simulink model "I_Control_and_G_Control_and_B_Control"  (R2024b)
settings: Solver=VariableStepAuto  StartTime=0.0  StopTime=time  RelTol=1e-3
values from neighbouring files (symbols this model uses):
  B = (y1-y4)/2    (= 0.75)    [Data.m]
  Cd = 0.28    [Data.m]
  dd = 2    [Data.m]
  delay_Pulse_time = 1.5    [Data.m]
  dk = 2    [Data.m]
  Fi = Ti/r    (= 156.25)    [Data.m]
  Fz = la/(la+lb)*m*g/2    (= 2450)    [Data.m]
  id = 0.01    [Data.m]
  ik = 1    [Data.m]
  Iw = 0.5    [Data.m]
  Iz = 1600    [Data.m]
  JL = 0.08    [Data.m]
  Jm = 6.96e-6    (= 6.96e-06)    [Data.m]
  Kb = 0.0525    [Data.m]
  Kf = 1.4e-3    (= 0.0014)    [Data.m]
  Km = 0.053    [Data.m]
  L = 6.2e-4    (= 0.00062)    [Data.m]    (also in submit.m = (1-nameda1)*(1-0.015*u1*sqrt((cx^2)*(nameda1^2)+(cy^2)*((tan)
  la = x1    (= 1.25)    [Data.m]
  lb = x1    (= 1.25)    [Data.m]
  m = 1000    [Data.m]
  n = 1/200    (= 0.005)    [Data.m]
  pd = 100    [Data.m]
  pk = 300    [Data.m]
  r = 0.32    [Data.m]
  R = 2.07    [Data.m]
  x1_fc = 0.01    [Data.m]
  x1_jz = 0    [Data.m]
  x2_fc = 0.05    [Data.m]
  x2_jz = 0.01    [Data.m]
  x3_fc = 0.1    [Data.m]
  x3_jz = 0.05    [Data.m]
  x4_fc = 0.5    [Data.m]
  x4_jz = 0.08    [Data.m]
  Xicr = 0,Yicr=10    [Data.m]
undefined symbols (not defined in the file or in its folder): Yicr
libraries: slpidlib x8
settings Model: Creator=hzh  LastModifiedBy=hzh
settings DataIOCC: ReturnWorkspaceOutputsName=out2
settings RTWCC: GPUComputeCapability=3.5

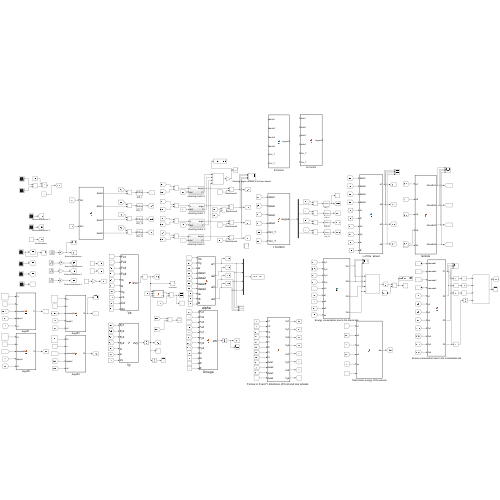
[thumbnail: Simulink's stored preview of the top-level diagram]
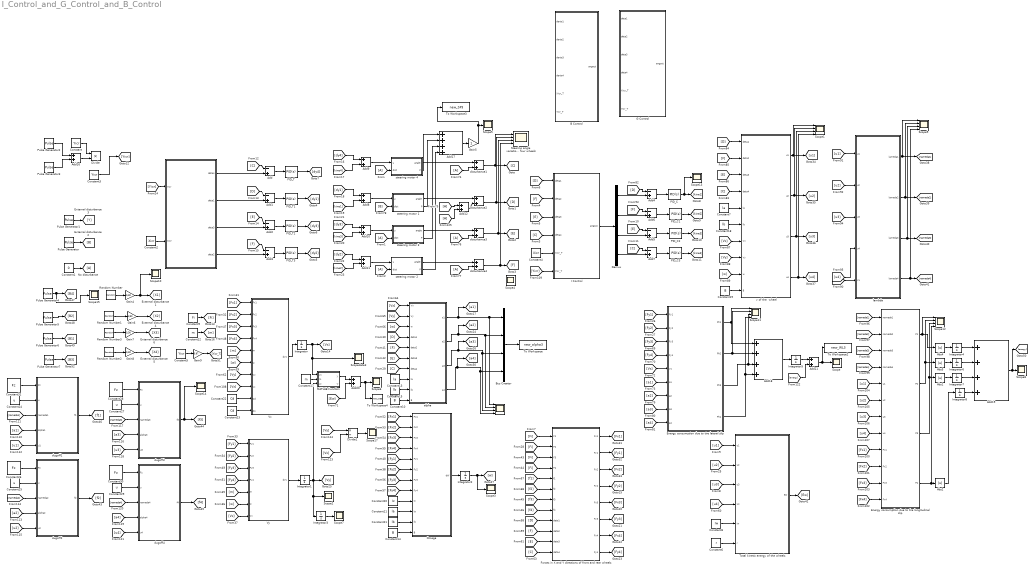
== system I_Control_and_G_Control_and_B_Control ==
  " " : MATLAB Function  TreatAsAtomicUnit=on
  "                    " : Scope  NumInputPorts=4
  Abs{1..2,4..5} (4 alike) : Abs  SaturateOnIntegerOverflow=off
  Add{,1..7} (8 alike) : Sum  Inputs=-+
  Add{8..12,16,20..21} (8 alike) : Sum
  Add17 : Sum  Inputs=++++
  Add18 : Sum  Inputs=++++
  Add19 : Sum  Inputs=++++
  B Control : MATLAB Function  TreatAsAtomicUnit=on
  Bus Creator : BusCreator  Inputs=4
  Constant : Constant  Value=Yicr
  Constant1 : Constant  Value=0
  Constant10 : Constant  Value=B
  Constant11 : Constant  Value=la
  Constant12 : Constant  Value=m
  Constant13 : Constant  Value=la
  Constant14 : Constant  Value=B
  Constant15 : Constant  Value=lb
  Constant17 : Constant  Value=m
  Constant18 : Constant  Value=lb
  Constant19 : Constant  Value=B
  Constant2 : Constant  Value=Xicr
  Constant20 : Constant  Value=Iz
  Constant21 : Constant  Value=lb
  Constant22 : Constant  Value=Cd
  Constant23 : Constant  Value=Cd
  Constant{24..25,27,29} (4 alike) : Constant  Value=u
  Constant{26,28,30..31} (4 alike) : Constant  Value=Fz
  Constant3 : Constant  Value=Yicr
  Constant4 : Constant  Value=Xicr
  Constant5 : Constant  Value=Yicr
  Constant6 : Constant  Value=r
  Constant7 : Constant  Value=la
  Constant8 : Constant  Value=Iw
  Constant9 : Constant  Value=Fi
  Demux : Demux
  Divide : Product  Inputs=**
  Divide1 : Product  Inputs=*/
  Energy consumption due to tire lateral slip : MATLAB Function  TreatAsAtomicUnit=on
  Energy consumption due to tire longitudinal slip : MATLAB Function  TreatAsAtomicUnit=on
  "Forces in X and Y directions of front and rear wheels  " : MATLAB Function  TreatAsAtomicUnit=on
  From{,1..2,74..77,125} (8 alike) : From
  G Control : MATLAB Function  TreatAsAtomicUnit=on
  Gain{4,6..8} (4 alike) : Gain  Gain=1/30
  Gain5 : Gain
  Gain9 : Gain  Gain=0.97
  I Control : MATLAB Function  TreatAsAtomicUnit=on
  Integrator : Integrator  InitialCondition=0.0001
  Integrator1 : Integrator
  Integrator2 : Integrator
  Integrator3 : Integrator
  Integrator{4..8} (5 alike) : Integrator  InitialCondition=0.01
  MATLAB Function : MATLAB Function  TreatAsAtomicUnit=on
  No disturbance : Goto
  Omega : MATLAB Function  TreatAsAtomicUnit=on
  PID_C{,1..3} (4 alike) : slpidlib/PID Controller  Controller=PID  Form=Parallel  TimeDomain=Continuous-time  UseExternalTs=off  SampleTime=-1  IntegratorMethod=Forward Euler  FilterMethod=Forward Euler  ControllerParametersSource=internal  P=pk  I=ik  UseKiTs=off  D=dk  UseExternalDerivativeSource=off  N=100  UseFilter=on  TunerSelectOption=Transfer Function Based (PID Tuner App)  InitialConditionSource=internal  InitialConditionForIntegrator=0  InitialConditionForFilter=0  DifferentiatorICPrevScaledInput=0  ExternalReset=none  TrackingMode=off  Kt=1  LimitOutput=off  SatLimitsSource=internal  UpperSaturationLimit=inf  LowerSaturationLimit=-inf  LinearizeAsGain=on  AntiWindupMode=none  Kb=1  LimitIntegrator=off  UpperIntegratorSaturationLimit=inf  LowerIntegratorSaturationLimit=-inf  POutMin=[]  POutMax=[]  IOutMin=[]  IOutMax=[]  DOutMin=[]  DOutMax=[]  NOutMin=[]  NOutMax=[]  SumOutMin=[]  SumOutMax=[]  SaturationOutMin=[]  SaturationOutMax=[]  PParamMin=[]  PParamMax=[]  IParamMin=[]  IParamMax=[]  DParamMin=[]  DParamMax=[]  NParamMin=[]  NParamMax=[]  KbParamMin=[]  KbParamMax=[]  KtParamMin=[]  KtParamMax=[]  KbOutMin=[]  KbOutMax=[]  KtOutMin=[]  KtOutMax=[]  IntegratorOutMin=[]  IntegratorOutMax=[]  FilterOutMin=[]  FilterOutMax=[]  SumI1OutMin=[]  SumI1OutMax=[]  SumI2OutMin=[]  SumI2OutMax=[]  SumI3OutMin=[]  SumI3OutMax=[]  SumI4OutMin=[]  SumI4OutMax=[]  SumDOutMin=[]  SumDOutMax=[]  DifferentiatorOutMin=[]  DifferentiatorOutMax=[]  FilterDiffOutCoefMin=[]  FilterDiffOutCoefMax=[]  ReciprocalOutMin=[]  ReciprocalOutMax=[]  SumDenOutMin=[]  SumDenOutMax=[]  SumNumOutMin=[]  SumNumOutMax=[]  DivideOutMin=[]  DivideOutMax=[]  UdiffTsProdOutMin=[]  UdiffTsProdOutMax=[]  NTsProdOutMin=[]  NTsProdOutMax=[]  UintegralTsProdOutMin=[]  UintegralTsProdOutMax=[]  UngainTsProdOutMin=[]  UngainTsProdOutMax=[]  ClampingZeroOutDataTypeStr=Inherit: Inherit via back propagation  ClampingZeroOutMin=[]  ClampingZeroOutMax=[]  FilterDenConstantOutDataTypeStr=Inherit: Inherit via back propagation  FilterDenConstantOutMin=[]  FilterDenConstantOutMax=[]  PCopyOutDataTypeStr=Inherit: Inherit via back propagation  PCopyOutMin=[]  PCopyOutMax=[]  NCopyOutDataTypeStr=Inherit: Inherit via back propagation  NCopyOutMin=[]  NCopyOutMax=[]  IntegratorContinuousStateAttributes=''  IntegratorStateMustResolveToSignalObject=off  IntegratorRTWStateStorageClass=Auto  FilterContinuousStateAttributes=''  FilterStateMustResolveToSignalObject=off  FilterRTWStateStorageClass=Auto  ParallelPVariant=InternalParameters  IdealPVariant=Disabled  IVariant=InternalParameters  DVariant=InternalParameters  IntegratorVariant=Continuous  SatVariant=Disabled  AWVariant=Passthrough  PCopyVariant=Disabled  TRVariant=Disabled  FdbkBlocksVariant=Forward  IdealPFdbkVariant=Disabled  SatFdbkVariant=Disabled  DerivativeFilterVariant=ContFilter  NVariant=InternalParameters  NCopyVariant=Disabled  FilterICVariant=InternalICsFilter  IntegratorICVariant=InternalICs  ExternalResetVariant=Disabled  TRSumVariant=Passthrough  SumFdbkVariant=Disabled  SumVariant=Sum_PID  TsampFilterVariant=InternalTs  TsampNgainVariant=Passthrough  TsampIntegralVariant=Disabled_SignalSpec  ExternalSaturationOutDataTypeStr=Inherit: Same as second input  DerivativeSourceVariant=ErrorSignal  PreIntVariant=InternalPreInt
  PID_T{,1..3} (4 alike) : slpidlib/PID Controller  Controller=PID  Form=Parallel  TimeDomain=Continuous-time  UseExternalTs=off  SampleTime=-1  IntegratorMethod=Forward Euler  FilterMethod=Forward Euler  ControllerParametersSource=internal  P=pd  I=id  UseKiTs=off  D=dd  UseExternalDerivativeSource=off  N=100  UseFilter=on  TunerSelectOption=Transfer Function Based (PID Tuner App)  InitialConditionSource=internal  InitialConditionForIntegrator=0  InitialConditionForFilter=0  DifferentiatorICPrevScaledInput=0  ExternalReset=none  TrackingMode=off  Kt=1  LimitOutput=off  SatLimitsSource=internal  UpperSaturationLimit=inf  LowerSaturationLimit=-inf  LinearizeAsGain=on  AntiWindupMode=none  Kb=1  LimitIntegrator=off  UpperIntegratorSaturationLimit=inf  LowerIntegratorSaturationLimit=-inf  POutMin=[]  POutMax=[]  IOutMin=[]  IOutMax=[]  DOutMin=[]  DOutMax=[]  NOutMin=[]  NOutMax=[]  SumOutMin=[]  SumOutMax=[]  SaturationOutMin=[]  SaturationOutMax=[]  PParamMin=[]  PParamMax=[]  IParamMin=[]  IParamMax=[]  DParamMin=[]  DParamMax=[]  NParamMin=[]  NParamMax=[]  KbParamMin=[]  KbParamMax=[]  KtParamMin=[]  KtParamMax=[]  KbOutMin=[]  KbOutMax=[]  KtOutMin=[]  KtOutMax=[]  IntegratorOutMin=[]  IntegratorOutMax=[]  FilterOutMin=[]  FilterOutMax=[]  SumI1OutMin=[]  SumI1OutMax=[]  SumI2OutMin=[]  SumI2OutMax=[]  SumI3OutMin=[]  SumI3OutMax=[]  SumI4OutMin=[]  SumI4OutMax=[]  SumDOutMin=[]  SumDOutMax=[]  DifferentiatorOutMin=[]  DifferentiatorOutMax=[]  FilterDiffOutCoefMin=[]  FilterDiffOutCoefMax=[]  ReciprocalOutMin=[]  ReciprocalOutMax=[]  SumDenOutMin=[]  SumDenOutMax=[]  SumNumOutMin=[]  SumNumOutMax=[]  DivideOutMin=[]  DivideOutMax=[]  UdiffTsProdOutMin=[]  UdiffTsProdOutMax=[]  NTsProdOutMin=[]  NTsProdOutMax=[]  UintegralTsProdOutMin=[]  UintegralTsProdOutMax=[]  UngainTsProdOutMin=[]  UngainTsProdOutMax=[]  ClampingZeroOutDataTypeStr=Inherit: Inherit via back propagation  ClampingZeroOutMin=[]  ClampingZeroOutMax=[]  FilterDenConstantOutDataTypeStr=Inherit: Inherit via back propagation  FilterDenConstantOutMin=[]  FilterDenConstantOutMax=[]  PCopyOutDataTypeStr=Inherit: Inherit via back propagation  PCopyOutMin=[]  PCopyOutMax=[]  NCopyOutDataTypeStr=Inherit: Inherit via back propagation  NCopyOutMin=[]  NCopyOutMax=[]  IntegratorContinuousStateAttributes=''  IntegratorStateMustResolveToSignalObject=off  IntegratorRTWStateStorageClass=Auto  FilterContinuousStateAttributes=''  FilterStateMustResolveToSignalObject=off  FilterRTWStateStorageClass=Auto  ParallelPVariant=InternalParameters  IdealPVariant=Disabled  IVariant=InternalParameters  DVariant=InternalParameters  IntegratorVariant=Continuous  SatVariant=Disabled  AWVariant=Passthrough  PCopyVariant=Disabled  TRVariant=Disabled  FdbkBlocksVariant=Forward  IdealPFdbkVariant=Disabled  SatFdbkVariant=Disabled  DerivativeFilterVariant=ContFilter  NVariant=InternalParameters  NCopyVariant=Disabled  FilterICVariant=InternalICsFilter  IntegratorICVariant=InternalICs  ExternalResetVariant=Disabled  TRSumVariant=Passthrough  SumFdbkVariant=Disabled  SumVariant=Sum_PID  TsampFilterVariant=InternalTs  TsampNgainVariant=Passthrough  TsampIntegralVariant=Disabled_SignalSpec  ExternalSaturationOutDataTypeStr=Inherit: Same as second input  DerivativeSourceVariant=ErrorSignal  PreIntVariant=InternalPreInt
  Pulse Generator : DiscretePulseGenerator  PulseType=Time based  Amplitude=(Pulse)  Period=100  PulseWidth=0.2  PhaseDelay=delay_Pulse_time
  Pulse Generator1 : DiscretePulseGenerator  PulseType=Time based  Amplitude=50  Period=100  PulseWidth=0.2  PhaseDelay=4
  Pulse Generator2 : DiscretePulseGenerator  PulseType=Time based  Period=5  PulseWidth=50
  Pulse Generator3 : DiscretePulseGenerator  PulseType=Time based  Amplitude=-1  Period=5  PulseWidth=50  PhaseDelay=2.5
  Pulse Generator4 : DiscretePulseGenerator  PulseType=Time based  Amplitude=0.16  Period=15  PulseWidth=15  PhaseDelay=12
  Pulse Generator5 : DiscretePulseGenerator  PulseType=Time based  Amplitude=0.1  Period=15  PulseWidth=5  PhaseDelay=8
  Pulse Generator6 : DiscretePulseGenerator  PulseType=Time based  Amplitude=0.05  Period=10  PulseWidth=5  PhaseDelay=4
  Pulse Generator7 : DiscretePulseGenerator  PulseType=Time based  Amplitude=0.2  Period=15  PulseWidth=4  PhaseDelay=1.5
  Random Number : RandomNumber  Mean=x1_jz  Variance=x1_fc  SampleTime=0.1
  Random Number1 : RandomNumber  Mean=x2_jz  Variance=x2_fc  SampleTime=0.1
  Random Number2 : RandomNumber  Mean=x4_jz  Variance=x4_fc  SampleTime=0.1
  Random Number3 : RandomNumber  Mean=x3_jz  Variance=x3_fc  SampleTime=0.1
  Scope{,2..3,5..8,10,13..15,17} (12 alike) : Scope
  Scope{1,9,11..12} (4 alike) : Scope  NumInputPorts=4
  Scope4 : Scope  NumInputPorts=2
  Scopedata3 : Scope
  Steering angle variation of the four wheels : Scope  NumInputPorts=4
  To Workspace : ToWorkspace  VariableName=new_alpha3  SampleTime=-1
  To Workspace2 : ToWorkspace  VariableName=new_WL3  SampleTime=-1
  To Workspace3 : ToWorkspace  VariableName=new_SP3  SampleTime=-1
  To Workspace4 : ToWorkspace  VariableName=new_KE3  SampleTime=-1
  Total kinetic energy of the wheels : MATLAB Function  TreatAsAtomicUnit=on
  Vx : MATLAB Function  TreatAsAtomicUnit=on
  Vy : MATLAB Function  TreatAsAtomicUnit=on
  alpha : MATLAB Function  TreatAsAtomicUnit=on
  disturbance{1..4} (4 alike) : Sum
  "dugoff1 " : MATLAB Function  TreatAsAtomicUnit=on
  dugoff2 : MATLAB Function  TreatAsAtomicUnit=on
  dugoff3 : MATLAB Function  TreatAsAtomicUnit=on
  dugoff4 : MATLAB Function  TreatAsAtomicUnit=on
  lambda : MATLAB Function  TreatAsAtomicUnit=on
  steering motor 1 : Subsystem
  steering motor 2 : Subsystem
  steering motor 3 : Subsystem
  steering motor 4 : Subsystem
  v of the  wheel : MATLAB Function  TreatAsAtomicUnit=on
  wires:
  Energy consumption due to tire longitudinal slip/2(P2) -> Abs5/1, Scope12/2
  " "/2(deta1) -> Add1/2
  [u3] -> Energy consumption due to tire longitudinal slip/7(u3)
  alpha/4(a4) -> [a4], "                    "/4, Bus Creator/4
  Integrator6/1 -> Add19/2
  " "/3(deta3) -> Add2/2
  [Fx4] -> Energy consumption due to tire longitudinal slip/12(Fx4)
  "Forces in X and Y directions of front and rear wheels  "/6(Fy3) -> [Fy3]
  Integrator8/1 -> Add19/4
  [Fx2] -> Energy consumption due to tire longitudinal slip/10(Fx2)
  Add6/1 -> PID_C1/1
  Abs4/1 -> Integrator4/1
  Demux/4 -> Add7/2
  Abs2/1 -> Integrator8/1
  Abs5/1 -> Integrator6/1
  [a4] -> Energy consumption due to tire lateral slip/9(a4)
  v of the  wheel/2(u2) -> Scope1/2, [u2]
  [Vx] -> alpha/1(Vx)
  [C] -> Add/1
  lambda/3(lameda3) -> [nameda3], Scope9/3
  [Fx3] -> Energy consumption due to tire longitudinal slip/11(Fx3)
  v of the  wheel/3(u3) -> Scope1/3, [u3]
  [Fi] -> "Forces in X and Y directions of front and rear wheels  "/1(F1)
  Energy consumption due to tire longitudinal slip/1(P1) -> Abs4/1, Scope12/1
  [a1] -> Energy consumption due to tire lateral slip/6(a1)
  Energy consumption due to tire longitudinal slip/3(P3) -> Abs1/1, Scope12/3
  From77/1 -> disturbance4/2
  Constant12/1 -> [m]
  Add18/1 -> Integrator5/1
  Add19/1 -> [energy], Scope8/1
  [u1] -> lambda/1(u1)
  Energy consumption due to tire lateral slip/4(Ph4) -> Add18/4, Scope11/4
  [u2] -> Energy consumption due to tire longitudinal slip/6(u2)
  [B] -> steering motor 1/2(dist)
  lambda/4(lameda4) -> Scope9/4, [nameda4]
  [nameda4] -> Energy consumption due to tire longitudinal slip/4(nameda4)
  [Vx] -> v of the  wheel/7(Vx)
  Energy consumption due to tire lateral slip/3(Ph3) -> Scope11/3, Add18/3
  lambda/2(lameda2) -> Scope9/2, [nameda2]
  [nameda2] -> Energy consumption due to tire longitudinal slip/2(nameda2)
  [w] -> Vx/6(w)
  Omega/1(dW) -> Integrator2/1
  Constant18/1 -> v of the  wheel/6(lb)
  Add11/1 -> steering motor 2/1(u)
  [a2] -> Energy consumption due to tire lateral slip/7(a2)
  [Fi] -> "Forces in X and Y directions of front and rear wheels  "/4(F4)
  steering motor 1/2(P) -> Add17/2
  [u4] -> lambda/4(u4)
  [F] -> v of the  wheel/2(deta2)
  Constant10/1 -> alpha/10(B)
  [kine4] -> Add9/2
  [u2] -> lambda/2(u2)
  Integrator7/1 -> Add19/3
  Integrator2/1 -> Scope3/1, [w]
  Constant7/1 -> v of the  wheel/5(la)
  [Yicr] -> " "/1(Yicr)
  [Vx] -> lambda/5(Vx)
  Energy consumption due to tire lateral slip/2(Ph2) -> Scope11/2, Add18/2
  [w] -> v of the  wheel/9(w)
  [D] -> v of the  wheel/1(deta1)
  [Vy] -> v of the  wheel/8(Vy)
  steering motor 4/2(P) -> Add17/1
  [a3] -> Energy consumption due to tire lateral slip/8(a3)
  PID_T3/1 -> [dy2]
  [Fy1] -> Energy consumption due to tire lateral slip/1(Fy1)
  [Fy3] -> Energy consumption due to tire lateral slip/3(Fy3)
  [Vx] -> Energy consumption due to tire lateral slip/5(Vx)
  [D] -> "Forces in X and Y directions of front and rear wheels  "/9(deta1)
  PID_C/1 -> Scope13/1, [kine1]
  Energy consumption due to tire lateral slip/1(Ph1) -> Scope11/1, Add18/1
  Integrator/1 -> [Vx], Scopedata3/1, MATLAB Function/1(vx)
  Constant2/1 -> " "/2(Xicr)
  [Fx1] -> Omega/1(Fx1)
  Add2/1 -> PID_T2/1
  "Forces in X and Y directions of front and rear wheels  "/3(Fx2) -> [Fx2]
  [f4] -> "Forces in X and Y directions of front and rear wheels  "/8(f4)
  Gain6/1 -> [X2]
  Constant13/1 -> alpha/8(la)
  [Fi] -> "Forces in X and Y directions of front and rear wheels  "/2(F2)
  Random Number3/1 -> Gain7/1
  Gain8/1 -> [X4]
  Gain7/1 -> [X3]
  [Fy2] -> Vy/2(Fy2)
  [u4] -> Energy consumption due to tire longitudinal slip/8(u4)
  Add17/1 -> Gain5/1
  [nameda3] -> Energy consumption due to tire longitudinal slip/3(nameda3)
  [Fy2] -> Omega/6(Fy2)
  [Fx2] -> Omega/2(Fx2)
  Random Number1/1 -> Gain6/1
  [E] -> v of the  wheel/3(deta3)
  Integrator3/1 -> Scope7/1
  Constant/1 -> Divide/1
  " "/1(deta4) -> Add/2
  PID_C2/1 -> [kine3]
  Add16/1 -> Divide/2
  From76/1 -> disturbance3/2
  [nameda1] -> Energy consumption due to tire longitudinal slip/1(nameda1)
  [D] -> Add4/1
  steering motor 2/1(angle) -> disturbance4/1
  v of the  wheel/1(u1) -> Scope1/1, [u1]
  PID_C1/1 -> [kine2]
  Gain5/1 -> To Workspace3/1, Scope5/1
  Constant20/1 -> Omega/9(Iz)
  [u3] -> lambda/3(u3)
  steering motor 2/2(P) -> Add17/4
  steering motor 3/2(P) -> Add17/3
  " "/4(deta2) -> Add3/2
  Demux/2 -> Add6/2
  Pulse Generator3/1 -> Add16/2
  [C] -> v of the  wheel/4(deta4)
  disturbance2/1 -> Steering angle variation of the four wheels/2, [D]
  disturbance3/1 -> Steering angle variation of the four wheels/3, [E]
  [Fx3] -> Vx/3(Fx3)
  [m] -> Vy/5(m)
  Integrator1/1 -> MATLAB Function/3(vy), Integrator3/1, Scope2/1, [Vy]
  Pulse Generator/1 -> [B]
  "Forces in X and Y directions of front and rear wheels  "/1(Fx1) -> [Fx1]
  Pulse Generator1/1 -> [Y]
  From74/1 -> disturbance1/2
  Constant11/1 -> Omega/10(la)
  [u1] -> Energy consumption due to tire longitudinal slip/5(u1)
  Random Number/1 -> Gain4/1
  [Fx4] -> Vx/4(Fx4)
  Vx/1(dVx) -> Integrator/1
  disturbance1/1 -> Steering angle variation of the four wheels/1, [C]
  "Forces in X and Y directions of front and rear wheels  "/5(Fx3) -> [Fx3]
  Vy/1(dVy) -> Integrator1/1
  Constant17/1 -> MATLAB Function/2(m)
  Gain4/1 -> Scope10/1, [X1]
  [Fx3] -> Omega/3(Fx3)
  [Fy4] -> Vy/4(Fy4)
  lambda/1(lameda1) -> Scope9/1, [nameda1]
  Constant21/1 -> Omega/11(lb)
  [Fy3] -> Vy/3(Fy3)
  [Vy] -> alpha/2(Vy)
  [Fy1] -> Omega/5(Fy1)
  [kine1] -> Add8/2
  Energy consumption due to tire longitudinal slip/4(P4) -> Abs2/1, Scope12/4
  [D] -> alpha/4(deta1)
  "Forces in X and Y directions of front and rear wheels  "/4(Fy2) -> [Fy2]
  Abs1/1 -> Integrator7/1
  [Fy3] -> Omega/7(Fy3)
  Constant14/1 -> Omega/12(B)
  [Fy4] -> Omega/8(Fy4)
  Constant19/1 -> v of the  wheel/10(B)
  [E] -> "Forces in X and Y directions of front and rear wheels  "/11(deta3)
  [Fx1] -> Vx/1(Fx1)
  [Vy] -> Vx/7(Vy)
  [Fy2] -> Energy consumption due to tire lateral slip/2(Fy2)
  [f2] -> "Forces in X and Y directions of front and rear wheels  "/6(f2)
  [w] -> alpha/3(w)
  [F] -> alpha/5(deta2)
  Integrator4/1 -> Add19/1
  [C] -> "Forces in X and Y directions of front and rear wheels  "/12(deta4)
  [E] -> alpha/6(deta3)
  [C] -> alpha/7(deta4)
  alpha/2(a2) -> Bus Creator/2, "                    "/2, [a2]
  "Forces in X and Y directions of front and rear wheels  "/8(Fy4) -> [Fy4]
  alpha/3(a3) -> Bus Creator/3, "                    "/3, [a3]
  [Vx] -> Vy/7(Vx)
  PID_T2/1 -> [dy3]
  [F] -> "Forces in X and Y directions of front and rear wheels  "/10(deta2)
  [m] -> Vx/5(m)
  [dy2] -> Add11/1
  [w] -> Vy/6(w)
  Constant9/1 -> [Fi]
  steering motor 3/1(angle) -> disturbance3/1
  Constant15/1 -> alpha/9(lb)
  [dy4] -> Add9/1
  Demux/1 -> Add4/2
  [Fx1] -> Energy consumption due to tire longitudinal slip/9(Fx1)
  [E] -> Add2/1
  Add8/1 -> steering motor 1/1(u)
  [f3] -> "Forces in X and Y directions of front and rear wheels  "/7(f3)
  [Fx4] -> Omega/4(Fx4)
  Add7/1 -> PID_C3/1
  Add10/1 -> steering motor 3/1(u)
  Constant1/1 -> No disturbance/1
  From1/1 -> steering motor 3/2(dist)
  From/1 -> steering motor 4/2(dist)
  [f1] -> "Forces in X and Y directions of front and rear wheels  "/5(f1)
  "Forces in X and Y directions of front and rear wheels  "/2(Fy1) -> [Fy1]
  PID_T1/1 -> [dy1]
  disturbance4/1 -> Steering angle variation of the four wheels/4, [F]
  [F] -> Add3/1
  [E] -> Add5/1
  [Fy4] -> Energy consumption due to tire lateral slip/4(Fy4)
  [dy1] -> Add8/1
  Add5/1 -> PID_C2/1
  Random Number2/1 -> Gain8/1
  [dy3] -> Add10/1
  [Fy1] -> Vy/1(Fy1)
  "Forces in X and Y directions of front and rear wheels  "/7(Fx4) -> [Fx4]
  Add3/1 -> PID_T3/1
  [Fx2] -> Vx/2(Fx2)
  Add/1 -> PID_T/1
  [kine3] -> Add10/2
  [D] -> Add1/1
  v of the  wheel/4(u4) -> Scope1/4, [u4]
  Add1/1 -> PID_T1/1
  Add9/1 -> steering motor 4/1(u)
  [Fi] -> "Forces in X and Y directions of front and rear wheels  "/3(F3)
  [kine2] -> Add11/2
  Demux/3 -> Add5/2
  Add4/1 -> PID_C/1
  PID_C3/1 -> [kine4]
  Pulse Generator2/1 -> Add16/1
  From2/1 -> steering motor 2/2(dist)
  PID_T/1 -> [dy4]
  Add20/1 -> To Workspace4/1, Scope6/1
  MATLAB Function/1(y) -> Add20/1
  [Ew] -> Add20/2
  [u1] -> Total kinetic energy of the wheels/1(u1)
  Constant8/1 -> Total kinetic energy of the wheels/5(Iw)
  [u3] -> Total kinetic energy of the wheels/3(u3)
  Total kinetic energy of the wheels/1(Ew) -> [Ew]
  Constant6/1 -> Total kinetic energy of the wheels/6(r)
  [u4] -> Total kinetic energy of the wheels/4(u4)
  [u2] -> Total kinetic energy of the wheels/2(u2)
  [Vx] -> Vx/8(vx)
  Constant22/1 -> Vx/9(Cd)
  Constant23/1 -> Vx/10(As)
  [a1] -> "dugoff1 "/4(alpha1)
  "dugoff1 "/1(f1) -> [f1]
  Constant30/1 -> dugoff4/1(Fz)
  dugoff2/1(f2) -> [f2]
  [nameda2] -> dugoff2/3(nameda2)
  [u4] -> dugoff4/5(u4)
  Constant31/1 -> "dugoff1 "/1(Fz)
  dugoff3/1(f3) -> [f3], Scope14/1
  [nameda3] -> dugoff3/3(nameda3)
  Constant25/1 -> dugoff2/2(u)
  Constant24/1 -> "dugoff1 "/2(u)
  dugoff4/1(f4) -> [f4]
  Constant27/1 -> dugoff3/2(u)
  [a2] -> dugoff2/4(alpha2)
  [u2] -> dugoff2/5(u2)
  [nameda4] -> dugoff4/3(nameda4)
  [u1] -> "dugoff1 "/5(u1)
  Constant29/1 -> dugoff4/2(u)
  Constant26/1 -> dugoff2/1(Fz)
  [u3] -> dugoff3/5(u3)
  [a4] -> dugoff4/4(alpha4)
  [nameda1] -> "dugoff1 "/3(nameda1)
  Constant28/1 -> dugoff3/1(Fz)
  [a3] -> dugoff3/4(alpha3)
  Pulse Generator4/1 -> Scope15/1, [B4]
  Pulse Generator5/1 -> [B2]
  Pulse Generator6/1 -> [B1]
  [energy] -> Add21/2
  Add21/1 -> To Workspace2/1, Scope/1
  Constant5/1 -> Gain9/1
  Gain9/1 -> [Yicr_T]
  Pulse Generator7/1 -> [B3]
  [Vy] -> Divide1/1
  [Vx] -> Divide1/2
  Divide1/1 -> Scope17/1
  I Control/1(angout) -> Demux/1
  [F] -> Add6/1
  [C] -> Add7/1
  [D] -> I Control/1(deta1)
  [F] -> I Control/2(deta2)
  [E] -> I Control/3(deta3)
  [C] -> I Control/4(deta4)
  Constant4/1 -> I Control/5(Xicr_T)
  [Yicr] -> I Control/6(Yicr_T)
  alpha/1(a1) -> "                    "/1, Bus Creator/1, [a1]
  Bus Creator/1 -> To Workspace/1
  Integrator5/1 -> Add21/1
  steering motor 4/1(angle) -> disturbance1/1
  steering motor 1/1(angle) -> disturbance2/1
  Add12/1 -> disturbance2/2
  From75/1 -> Add12/1
  From125/1 -> Add12/2
  Constant3/1 -> [Yicr]

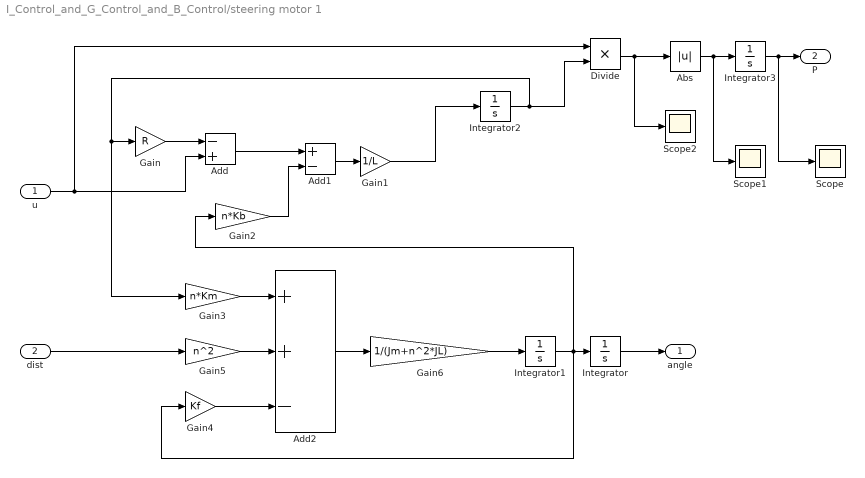
== system I_Control_and_G_Control_and_B_Control/steering motor 1 ==
  u : Inport
  dist : Inport  Port=2
  Abs : Abs  SaturateOnIntegerOverflow=off
  Add : Sum  Inputs=-+
  Add1 : Sum  Inputs=+-
  Add2 : Sum  Inputs=++-
  Divide : Product  Inputs=**
  Gain : Gain  Gain=R
  Gain1 : Gain  Gain=1/L
  Gain2 : Gain  Gain=n*Kb
  Gain3 : Gain  Gain=n*Km
  Gain4 : Gain  Gain=Kf
  Gain5 : Gain  Gain=n^2
  Gain6 : Gain  Gain=1/(Jm+n^2*JL)
  Integrator{,1..3} (4 alike) : Integrator
  Scope : Scope
  Scope1 : Scope
  Scope2 : Scope
  angle : Outport
  P : Outport  Port=2
  wires:
  Abs/1 -> Integrator3/1, Scope1/1
  Divide/1 -> Scope2/1, Abs/1
  Gain6/1 -> Integrator1/1
  Add2/1 -> Gain6/1
  Gain4/1 -> Add2/3
  Gain5/1 -> Add2/2
  Gain3/1 -> Add2/1
  dist/1 -> Gain5/1
  Gain1/1 -> Integrator2/1
  Add1/1 -> Gain1/1
  Gain2/1 -> Add1/2
  Add/1 -> Add1/1
  u/1 -> Add/2, Divide/1
  Gain/1 -> Add/1
  Integrator2/1 -> Divide/2, Gain/1, Gain3/1
  Integrator1/1 -> Integrator/1, Gain4/1, Gain2/1
  Integrator/1 -> angle/1
  Integrator3/1 -> P/1, Scope/1

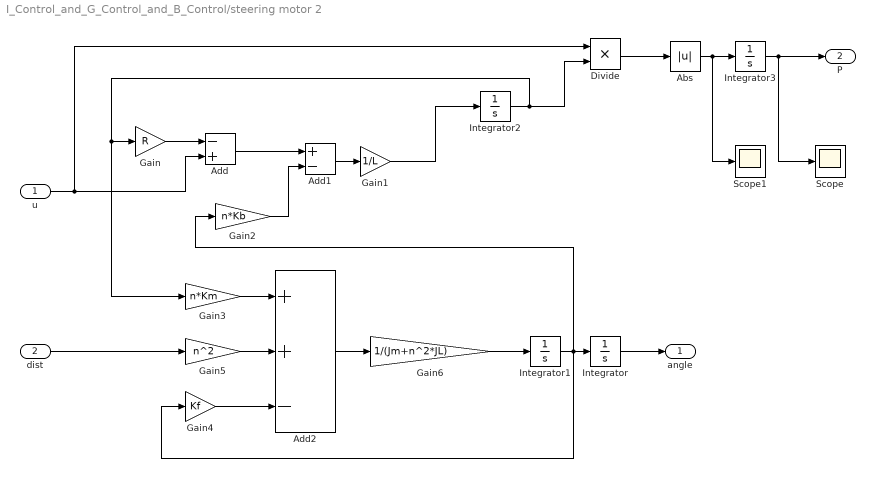
== system I_Control_and_G_Control_and_B_Control/steering motor 2 ==
  u : Inport
  dist : Inport  Port=2
  Abs : Abs  SaturateOnIntegerOverflow=off
  Add : Sum  Inputs=-+
  Add1 : Sum  Inputs=+-
  Add2 : Sum  Inputs=++-
  Divide : Product  Inputs=**
  Gain : Gain  Gain=R
  Gain1 : Gain  Gain=1/L
  Gain2 : Gain  Gain=n*Kb
  Gain3 : Gain  Gain=n*Km
  Gain4 : Gain  Gain=Kf
  Gain5 : Gain  Gain=n^2
  Gain6 : Gain  Gain=1/(Jm+n^2*JL)
  Integrator{,1..3} (4 alike) : Integrator
  Scope : Scope
  Scope1 : Scope
  angle : Outport
  P : Outport  Port=2
  wires:
  Abs/1 -> Integrator3/1, Scope1/1
  Divide/1 -> Abs/1
  Gain6/1 -> Integrator1/1
  Add2/1 -> Gain6/1
  Gain4/1 -> Add2/3
  Gain5/1 -> Add2/2
  Gain3/1 -> Add2/1
  dist/1 -> Gain5/1
  Gain1/1 -> Integrator2/1
  Add1/1 -> Gain1/1
  Gain2/1 -> Add1/2
  Add/1 -> Add1/1
  u/1 -> Add/2, Divide/1
  Gain/1 -> Add/1
  Integrator2/1 -> Divide/2, Gain/1, Gain3/1
  Integrator1/1 -> Integrator/1, Gain4/1, Gain2/1
  Integrator/1 -> angle/1
  Integrator3/1 -> P/1, Scope/1

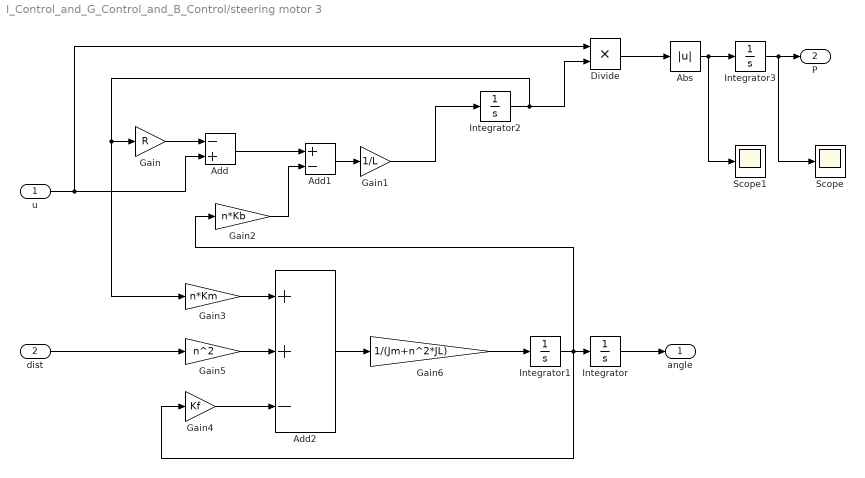
== system I_Control_and_G_Control_and_B_Control/steering motor 3 ==
  u : Inport
  dist : Inport  Port=2
  Abs : Abs  SaturateOnIntegerOverflow=off
  Add : Sum  Inputs=-+
  Add1 : Sum  Inputs=+-
  Add2 : Sum  Inputs=++-
  Divide : Product  Inputs=**
  Gain : Gain  Gain=R
  Gain1 : Gain  Gain=1/L
  Gain2 : Gain  Gain=n*Kb
  Gain3 : Gain  Gain=n*Km
  Gain4 : Gain  Gain=Kf
  Gain5 : Gain  Gain=n^2
  Gain6 : Gain  Gain=1/(Jm+n^2*JL)
  Integrator{,1..3} (4 alike) : Integrator
  Scope : Scope
  Scope1 : Scope
  angle : Outport
  P : Outport  Port=2
  wires:
  Integrator/1 -> angle/1
  Integrator1/1 -> Gain2/1, Gain4/1, Integrator/1
  Integrator2/1 -> Gain3/1, Gain/1, Divide/2
  Gain/1 -> Add/1
  u/1 -> Divide/1, Add/2
  Add/1 -> Add1/1
  Gain2/1 -> Add1/2
  Add1/1 -> Gain1/1
  Gain1/1 -> Integrator2/1
  dist/1 -> Gain5/1
  Gain3/1 -> Add2/1
  Gain5/1 -> Add2/2
  Gain4/1 -> Add2/3
  Add2/1 -> Gain6/1
  Gain6/1 -> Integrator1/1
  Divide/1 -> Abs/1
  Abs/1 -> Integrator3/1, Scope1/1
  Integrator3/1 -> P/1, Scope/1

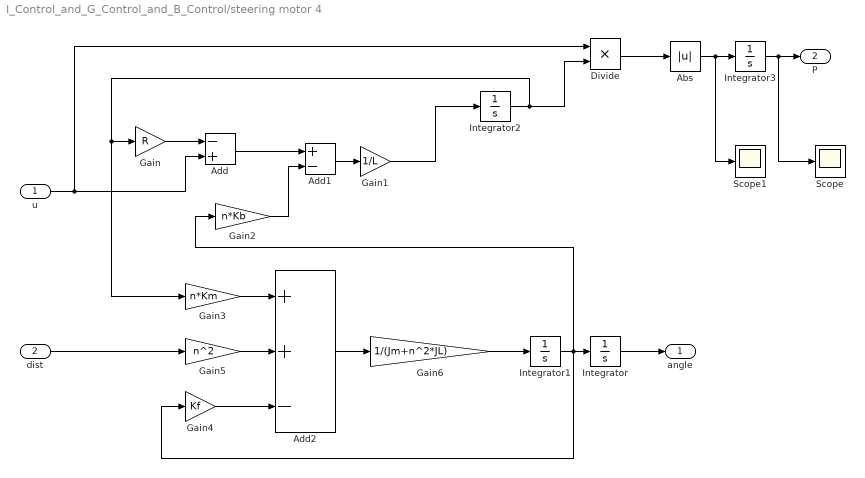
== system I_Control_and_G_Control_and_B_Control/steering motor 4 ==
  u : Inport
  dist : Inport  Port=2
  Abs : Abs  SaturateOnIntegerOverflow=off
  Add : Sum  Inputs=-+
  Add1 : Sum  Inputs=+-
  Add2 : Sum  Inputs=++-
  Divide : Product  Inputs=**
  Gain : Gain  Gain=R
  Gain1 : Gain  Gain=1/L
  Gain2 : Gain  Gain=n*Kb
  Gain3 : Gain  Gain=n*Km
  Gain4 : Gain  Gain=Kf
  Gain5 : Gain  Gain=n^2
  Gain6 : Gain  Gain=1/(Jm+n^2*JL)
  Integrator{,1..3} (4 alike) : Integrator
  Scope : Scope
  Scope1 : Scope
  angle : Outport
  P : Outport  Port=2
  wires:
  Integrator/1 -> angle/1
  Integrator1/1 -> Gain2/1, Gain4/1, Integrator/1
  Integrator2/1 -> Gain3/1, Gain/1, Divide/2
  Gain/1 -> Add/1
  u/1 -> Divide/1, Add/2
  Add/1 -> Add1/1
  Gain2/1 -> Add1/2
  Add1/1 -> Gain1/1
  Gain1/1 -> Integrator2/1
  dist/1 -> Gain5/1
  Gain3/1 -> Add2/1
  Gain5/1 -> Add2/2
  Gain4/1 -> Add2/3
  Add2/1 -> Gain6/1
  Gain6/1 -> Integrator1/1
  Divide/1 -> Abs/1
  Abs/1 -> Integrator3/1, Scope1/1
  Integrator3/1 -> P/1, Scope/1

== matlab function I_Control_and_G_Control_and_B_Control/Vx ==
  data: Fx1 input; dVx output; Fx2 input; Fx3 input; Fx4 input; m input; w input; Vy input; vx input; Cd input; As input
function dVx= fcn(Fx1,Fx2,Fx3,Fx4,m,w,Vy,vx,Cd,As)


dVx=(Fx1+Fx2+Fx3+Fx4-As*Cd*vx^2/21.15)/m+Vy*w;

== matlab function I_Control_and_G_Control_and_B_Control/v of the  wheel ==
  data: deta1 input; u1 output; deta2 input; deta3 input; deta4 input; la input; lb input; Vx input; Vy input; w input; B input; u2 output; u3 output; u4 output
function [u1,u2,u3,u4] = fcn(deta1,deta2,deta3,deta4,la,lb,Vx,Vy,w,B)

u1=(Vx-w*B)*cos(deta1)+(Vy+w*la)*sin(deta1);
u2=(Vx-w*B)*cos(deta2)+(Vy-w*lb)*sin(deta2);
u3=(Vx+w*B)*cos(deta3)+(Vy-w*lb)*sin(deta3);
u4=(Vx+w*B)*cos(deta4)+(Vy+w*la)*sin(deta4);

== matlab function I_Control_and_G_Control_and_B_Control/Energy consumption due to tire lateral slip ==
  data: Fy1 input; Ph1 output; Fy2 input; Fy3 input; Fy4 input; Vx input; a1 input; a2 input; a3 input; a4 input; Ph2 output; Ph3 output; Ph4 output
function [Ph1,Ph2,Ph3,Ph4] = fcn(Fy1,Fy2,Fy3,Fy4,Vx,a1,a2,a3,a4)

Ph1=-Fy1*Vx*a1;
Ph2=-Fy2*Vx*a2;
Ph3=-Fy3*Vx*a3;
Ph4=-Fy4*Vx*a4;

== matlab function I_Control_and_G_Control_and_B_Control/Energy consumption due to tire longitudinal slip ==
  data: nameda1 input; P1 output; nameda2 input; nameda3 input; nameda4 input; u1 input; u2 input; u3 input; u4 input; Fx1 input; Fx2 input; Fx3 input; Fx4 input; P2 output; P3 output; P4 output
function [P1,P2,P3,P4] = fcn(nameda1,nameda2,nameda3,nameda4,u1,u2,u3,u4,Fx1,Fx2,Fx3,Fx4)

P1=Fx1*nameda1*u1;
P2=Fx2*nameda2*u2;
P3=Fx3*nameda3*u3;
P4=Fx4*nameda4*u4;

== matlab function I_Control_and_G_Control_and_B_Control/MATLAB Function ==
  data: vx input; m input; vy input; y output; V output
function [y,V] = fcn(vx,m,vy)

y = 1/2*(sqrt(vx^2+vy^2))^2*m;
V=sqrt(vx^2+vy^2);

== matlab function I_Control_and_G_Control_and_B_Control/I Control ==
  data: deta1 input; angout output; deta2 input; deta3 input; deta4 input; Xicr_T input; Yicr_T input
function angout = fcn(deta1,deta2,deta3,deta4,Xicr_T,Yicr_T) %质心

a=[0,0,0,0];
b=[0,0,0,0];
x=[1.25,-1.25,-1.25,1.25];
y=[0.75,0.75,-0.75,-0.75];
angin=[deta1,deta2,deta3,deta4];
angout=[0,0,0,0];


if (abs(angin(1))>=0.001) && (abs(angin(2))>=0.001) && (abs(angin(3))>=0.001) && (abs(angin(4))>=0.001)
    for i=1:4
        a(i)=tan(angin(i)+pi/2)
        b(i)=y(i)-a(i)*x(i)
    end
    
   x1=-(b(1)-b(2))/(a(1)-a(2));
   y1=(a(1)*b(2)-a(2)*b(1))/(a(1)-a(2));

   x2=-(b(1)-b(3))/(a(1)-a(3));
   y2=(a(1)*b(3)-a(3)*b(1))/(a(1)-a(3));

   x3=-(b(4)-b(2))/(a(4)-a(2));
   y3=(a(4)*b(2)-a(2)*b(4))/(a(4)-a(2));

   x4=-(b(4)-b(3))/(a(4)-a(3));
   y4=(a(4)*b(3)-a(3)*b(4))/(a(4)-a(3));

   Xicr_c=(x1+x2+x3+x4)/4*0.995;
   Yicr_c=(y1+y2+y3+y4)/4*0.995;


    for i=1:4
        k=sign(angin(i)-atan2(y(i)-Yicr_c,x(i)-Xicr_c))
        angout(i)=atan2(k*(x(i)-Xicr_c),-k*(y(i)-Yicr_c))
    end
else
   angout=angin
end


% for i=1:4
%    a(i)=tan(angin(i)+pi/2);
%    b(i)=y(i)-a(i)*x(i);
% end
% 
% Xf=-(b(1)-b(4))/(a(1)-a(4));
% Yf=(a(1)*b(4)-a(4)*b(1))/(a(1)-a(4));
% Kf=Yf/(Xf-x(1));
% Bf=-Kf*x(1);
% 
% Xr=-(b(2)-b(3))/(a(2)-a(3));
% Yr=(a(2)*b(3)-a(3)*b(2))/(a(2)-a(3));
% Kr=Yr/(Xr-x(2));
% Br=-Kr*x(2);
% 
% Kz=Yicr_T/Xicr_T;
% Bz=0;
% 
% A=Bf*(Kr-Kz)*(Kr-Kf+Kz+Kf*Kr*Kz);
% B=Br*(Kz-Kf)*(Kz-Kr+Kf+Kf*Kr*Kz);
% C=Bz*(Kf-Kr)*(Kf-Kz+Kr+Kf*Kr*Kz);
% D=2*Xicr_T*(Kf-Kr)*(Kz-Kf)*(Kr-Kz);
% E=2*(Kr^2+1)*(Kf^2+1)*(Kz^2+1);
% 
% Xicr_c=(A+B+C+D)/E
% 
% F=Bf*(Kr-Kz)*(Kf*Kr+Kf*Kz-Kr*Kz+1);
% G=Bz*(Kf-Kr)*(Kf*Kz-Kf*Kr+Kr*Kz+1);
% H=Br*(Kz-Kf)*(Kf*Kr-Kf*Kz+Kr*Kz+1);
% I=2*Yicr_T*(Kf-Kr)*(Kf-Kz)*(Kr-Kz);
% 
% Yicr_c=-(F+G+H+I)/E
% 
% for i=1:4
%     k=sign(angin(i)-atan2(y(i)-Yicr_c,x(i)-Xicr_c));
%     angout(i)=atan2(k*(x(i)-Xicr_c),-k*(y(i)-Yicr_c));
% end

== matlab function I_Control_and_G_Control_and_B_Control/B Control ==
  data: derta1 input; angout output; derta2 input; derta3 input; derta4 input; Xicr_T input; Yicr_T input
function angout  = fcn(derta1,derta2,derta3,derta4,Xicr_T,Yicr_T) % B control

angin=[derta1,derta2,derta3,derta4];
angout=[0,0,0,0];
Xicr_c=0;
Yicr_c=0;

model=1
x=[1.25,-1.25,-1.25,1.25];
y=[0.75,0.75,-0.75,-0.75];
a=[0,0,0,0];
b=[0,0,0,0];

A1=0;
A2=0;
A3=0;
A4=0;
A5=0;

if model>0

    if angin(1)==angin(2) && angin(3)==angin(4) && angin(1)==angin(3)
        angout=angin;
    
    else
        for i=1:4
            a(i)=tan(angin(i)+pi/2)
            b(i)=y(i)-a(i)*x(i)
        end
       
        for i=1:4
            A1=A1+2*a(i)^2/(a(i)^2+1)
            A2=A2+2*a(i)/(a(i)^2+1)
            A3=A3+2*a(i)*b(i)/(a(i)^2+1)
            A4=A4+2/(a(i)^2+1)
            A5=A5+2*b(i)/(a(i)^2+1)
        end
       
        Xicr_c=(A2*A5-A3*A4)/(A1*A4-A2^2)
        Yicr_c=(A1*A5-A3*A2)/(A1*A4-A2^2)
        
        % Xicr_c=(Xicr_c+Xicr)/2;
        % Yicr_c=(Yicr_c+Yicr)/2;

        for i=1:4
            k=sign(angin(i)-atan2(y(i)-Yicr_c,x(i)-Xicr_c))
            angout(i)=atan2(k*(x(i)-Xicr_c),-k*(y(i)-Yicr_c))
        end
    end

else
    for i=1:4
            a(i)=tan(angin(i)+pi/2)
            b(i)=y(i)-a(i)*x(i)
        end

        for i=1:4
            A1=A1+2*a(i)^2/(a(i)^2+1)
            A2=A2+2*a(i)/(a(i)^2+1)
            A3=A3+2*a(i)*b(i)/(a(i)^2+1)
            A4=A4+2/(a(i)^2+1)
            A5=A5+2*b(i)/(a(i)^2+1)
        end

        Xicr_c=(A2*A5-A3*A4)/(A1*A4-A2^2)
        Yicr_c=(A1*A5-A3*A2)/(A1*A4-A2^2)
        sum2=0;
        for i=1:4
            sum2=sum2+angin(i);
        end

        for i=1:4
            angout(i)=sum2/4;
        end

end

== matlab function I_Control_and_G_Control_and_B_Control/Total kinetic energy of the wheels ==
  data: u1 input; Ew output; u2 input; u3 input; u4 input; Iw input; r input
function Ew = fcn(u1,u2,u3,u4,Iw,r)

Ew=1/2*Iw*((u1/r)^2+(u2/r)^2+(u3/r)^2+(u4/r)^2)

== matlab function I_Control_and_G_Control_and_B_Control/dugoff1  ==
  data: Fz input; u input; nameda1 input; alpha1 input; f1 output; u1 input
function f1 = tire(Fz,u,nameda1,alpha1,u1)
nameda1 = -nameda1;
cx = -4;
cy = -20;
L = (1-nameda1)*(1-0.015*u1*sqrt((cx^2)*(nameda1^2)+(cy^2)*((tan(alpha1))^2)))/(2*sqrt((cx^2)*(nameda1^2)+(cy^2)*((tan(alpha1))^2)));
if L<1
    fL = L*(2-L);
else
    fL = 1;
end
Fx0 = Fz*cx*nameda1*fL/(1-nameda1);
Fy0 = Fz*cy*tan(alpha1)*fL/(1-nameda1);
Fx = u*Fx0;
f1 = u*Fy0;

== matlab function I_Control_and_G_Control_and_B_Control/dugoff2 ==
  data: Fz input; u input; nameda2 input; alpha2 input; f2 output; u2 input
function f2 = tire(Fz,u,nameda2,alpha2,u2)
nameda2 = -nameda2;
cx = -4;
cy = -20;
L = (1-nameda2)*(1-0.015*u2*sqrt((cx^2)*(nameda2^2)+(cy^2)*((tan(alpha2))^2)))/(2*sqrt((cx^2)*(nameda2^2)+(cy^2)*((tan(alpha2))^2)));
if L<1
    fL = L*(2-L);
else
    fL = 1;
end
Fx0 = Fz*cx*nameda2*fL/(1-nameda2);
Fy0 = Fz*cy*tan(alpha2)*fL/(1-nameda2);
Fx = u*Fx0;
f2 = u*Fy0;

== matlab function I_Control_and_G_Control_and_B_Control/dugoff3 ==
  data: Fz input; u input; nameda3 input; alpha3 input; f3 output; u3 input
function f3 = tire(Fz,u,nameda3,alpha3,u3)
nameda3 = -nameda3;
cx = -4;
cy = -20;
L = (1-nameda3)*(1-0.015*u3*sqrt((cx^2)*(nameda3^2)+(cy^2)*((tan(alpha3))^2)))/(2*sqrt((cx^2)*(nameda3^2)+(cy^2)*((tan(alpha3))^2)));
if L<1
    fL = L*(2-L);
else
    fL = 1;
end
Fx0 = Fz*cx*nameda3*fL/(1-nameda3);
Fy0 = Fz*cy*tan(alpha3)*fL/(1-nameda3);
Fx = u*Fx0;
f3 = u*Fy0;

== matlab function I_Control_and_G_Control_and_B_Control/lambda ==
  data: u1 input; lameda1 output; u2 input; u3 input; u4 input; Vx input; lameda2 output; lameda3 output; lameda4 output
function [lameda1,lameda2,lameda3,lameda4] = fcn(u1,u2,u3,u4,Vx)

lameda1=(Vx-u1)/Vx;
lameda2=(Vx-u2)/Vx;
lameda3=(Vx-u3)/Vx;
lameda4=(Vx-u4)/Vx;

== matlab function I_Control_and_G_Control_and_B_Control/dugoff4 ==
  data: Fz input; u input; nameda4 input; alpha4 input; f4 output; u4 input
function f4 = tire(Fz,u,nameda4,alpha4,u4)
nameda4 = -nameda4;
cx = -4;
cy = -20;
L = (1-nameda4)*(1-0.015*u4*sqrt((cx^2)*(nameda4^2)+(cy^2)*((tan(alpha4))^2)))/(2*sqrt((cx^2)*(nameda4^2)+(cy^2)*((tan(alpha4))^2)));
if L<1
    fL = L*(2-L);
else
    fL = 1;
end
Fx0 = Fz*cx*nameda4*fL/(1-nameda4);
Fy0 = Fz*cy*tan(alpha4)*fL/(1-nameda4);
Fx = u*Fx0;
f4 = u*Fy0;

== matlab function I_Control_and_G_Control_and_B_Control/  ==
  data: Yicr input; deta4 output; deta1 output; deta3 output; deta2 output; Xicr input
function [deta4,deta1,deta3,deta2] = fcn(Yicr,Xicr)

x=[1.25,-1.25,-1.25,1.25];
y=[0.75,0.75,-0.75,-0.75];

if Yicr>0
    u1=1
    deta1=atan2(u1*(x(1)-Xicr),-u1*(y(1)-Yicr));
    deta2=atan2(u1*(x(2)-Xicr),-u1*(y(2)-Yicr));
    deta3=atan2(u1*(x(3)-Xicr),-u1*(y(3)-Yicr));
    deta4=atan2(u1*(x(4)-Xicr),-u1*(y(4)-Yicr));
else
    u1=-1
    deta1=atan2(u1*(x(1)-Xicr),-u1*(y(1)-Yicr));
    deta2=atan2(u1*(x(2)-Xicr),-u1*(y(2)-Yicr));
    deta3=atan2(u1*(x(3)-Xicr),-u1*(y(3)-Yicr));
    deta4=atan2(u1*(x(4)-Xicr),-u1*(y(4)-Yicr));
end

== matlab function I_Control_and_G_Control_and_B_Control/G Control ==
  data: deta1 input; angout output; deta2 input; deta3 input; deta4 input; Xicr_T input; Yicr_T input
function angout = fcn(deta1,deta2,deta3,deta4,Xicr_T,Yicr_T) %两轴线交点

a=[0,0,0,0];
b=[0,0,0,0];
x=[1.25,-1.25,-1.25,1.25];
y=[0.75,0.75,-0.75,-0.75];
angin=[deta1,deta2,deta3,deta4];
angout=[0,0,0,0];


if (abs(angin(1))>=0.001) && (abs(angin(2))>=0.001) && (abs(angin(3))>=0.001) && (abs(angin(4))>=0.001)
    for i=1:4
        a(i)=tan(angin(i)+pi/2)
        b(i)=y(i)-a(i)*x(i)
    end
    
    Xf=-(b(1)-b(4))/(a(1)-a(4))
    Yf=(a(1)*b(4)-a(4)*b(1))/(a(1)-a(4))
    Kf=Yf/(Xf-x(1))
    Bf=-Kf*x(1)

    Xr=-(b(2)-b(3))/(a(2)-a(3))
    Yr=(a(2)*b(3)-a(3)*b(2))/(a(2)-a(3))
    Kr=Yr/(Xr-x(2))
    Br=-Kr*x(2)

    Xicr_c=-(Bf-Br)/(Kf-Kr);
    Yicr_c=(Kf*Br-Kr*Bf)/(Kf-Kr);


    for i=1:4
        k=sign(angin(i)-atan2(y(i)-Yicr_c,x(i)-Xicr_c))
        angout(i)=atan2(k*(x(i)-Xicr_c),-k*(y(i)-Yicr_c))
    end
else
   angout=angin
end



% for i=1:4
%    a(i)=tan(angin(i)+pi/2);
%    b(i)=y(i)-a(i)*x(i);
% end
% 
% Xf=-(b(1)-b(4))/(a(1)-a(4));
% Yf=(a(1)*b(4)-a(4)*b(1))/(a(1)-a(4));
% Kf=Yf/(Xf-x(1));
% Bf=-Kf*x(1);
% 
% Xr=-(b(2)-b(3))/(a(2)-a(3));
% Yr=(a(2)*b(3)-a(3)*b(2))/(a(2)-a(3));
% Kr=Yr/(Xr-x(2));
% Br=-Kr*x(2);
% 
% Kz=Yicr_T/Xicr_T;
% Bz=0;
% 
% A=Bf*(Kr-Kz)*(Kr-Kf+Kz+Kf*Kr*Kz);
% B=Br*(Kz-Kf)*(Kz-Kr+Kf+Kf*Kr*Kz);
% C=Bz*(Kf-Kr)*(Kf-Kz+Kr+Kf*Kr*Kz);
% D=2*Xicr_T*(Kf-Kr)*(Kz-Kf)*(Kr-Kz);
% E=2*(Kr^2+1)*(Kf^2+1)*(Kz^2+1);
% 
% Xicr_c=(A+B+C+D)/E
% 
% F=Bf*(Kr-Kz)*(Kf*Kr+Kf*Kz-Kr*Kz+1);
% G=Bz*(Kf-Kr)*(Kf*Kz-Kf*Kr+Kr*Kz+1);
% H=Br*(Kz-Kf)*(Kf*Kr-Kf*Kz+Kr*Kz+1);
% I=2*Yicr_T*(Kf-Kr)*(Kf-Kz)*(Kr-Kz);
% 
% Yicr_c=-(F+G+H+I)/E
% 
% for i=1:4
%     k=sign(angin(i)-atan2(y(i)-Yicr_c,x(i)-Xicr_c));
%     angout(i)=atan2(k*(x(i)-Xicr_c),-k*(y(i)-Yicr_c));
% end

== matlab function I_Control_and_G_Control_and_B_Control/alpha ==
  data: Vx input; a1 output; Vy input; w input; deta1 input; deta2 input; deta3 input; deta4 input; la input; lb input; a2 output; B input; a3 output; a4 output
function [a1,a2,a3,a4] = fcn(Vx,Vy,w,deta1,deta2,deta3,deta4,la,lb,B)


a1=atan((Vy+la*w)/(Vx-w*B))-deta1;
a2=atan((Vy-lb*w)/(Vx-w*B))-deta2;
a3=atan((Vy-la*w)/(Vx+w*B))-deta3;
a4=atan((Vy+la*w)/(Vx+w*B))-deta4;

== matlab function I_Control_and_G_Control_and_B_Control/Forces in X and Y directions of front and rear wheels   ==
  data: F1 input; Fx1 output; F2 input; F3 input; F4 input; f1 input; f2 input; f3 input; f4 input; deta1 input; deta2 input; Fy1 output; Fx2 output; Fy2 output; deta3 input; deta4 input; Fx3 output; Fy3 output; Fx4 output; Fy4 output
function [Fx1,Fy1,Fx2,Fy2,Fx3,Fy3,Fx4,Fy4]= fcn(F1,F2, F3,F4,f1,f2,f3,f4,deta1,deta2,deta3,deta4)

Fx1=F1*cos(deta1)-f1*sin(deta1);
Fy1=F1*sin(deta1)+f1*cos(deta1);


Fx2=F2*cos(deta2)+f2*sin(deta2);
Fy2=-F2*sin(deta2)+f2*cos(deta2);

Fx3=F3*cos(deta3)+f3*sin(deta3);
Fy3=-F3*sin(deta3)+f3*cos(deta3);

Fx4=F4*cos(deta4)-f4*sin(deta4);
Fy4=F4*sin(deta4)+f4*cos(deta4);

== matlab function I_Control_and_G_Control_and_B_Control/Vy ==
  data: Fy1 input; dVy output; Fy2 input; Fy3 input; Fy4 input; m input; w input; Vx input
function dVy= fcn(Fy1,Fy2,Fy3,Fy4,m,w,Vx)


dVy=(Fy2+Fy1+Fy3+Fy4)/m-Vx*w;

== matlab function I_Control_and_G_Control_and_B_Control/Omega ==
  data: Fx1 input; Fx2 input; Fx3 input; Fx4 input; Fy1 input; dW output; Fy2 input; Fy3 input; Fy4 input; Iz input; la input; lb input; B input
function dW= fcn(Fx1,Fx2,Fx3,Fx4,Fy1,Fy2,Fy3,Fy4,Iz,la,lb,B)

% dW=((Fy4+Fy1)*la-(Fy2+Fy3)*lb)/Iz;

dW=((Fy4+Fy1)*la-(Fy2+Fy3)*lb+(Fx4+Fx3)*B-(Fx1+Fx2)*B)/Iz;
